simulink model "system1_time"  (R2019b)
settings: Solver=VariableStepAuto  StartTime=0.0  StopTime=10.0  RelTol=1e-3
settings Model: Creator=davis  LastModifiedBy=davis

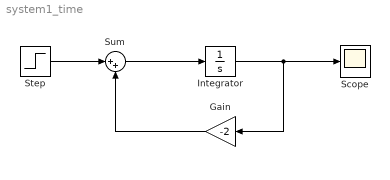
== system system1_time ==
  Gain : Gain  Gain=-2
  Integrator : Integrator  InitialCondition=1
  Scope : Scope
  Step : Step  Time=0  SampleTime=0
  Sum : Sum  Inputs=|++
  wires:
  Step/1 -> Sum/1
  Sum/1 -> Integrator/1
  Integrator/1 -> Gain/1, Scope/1
  Gain/1 -> Sum/2
